simulink model "Simulation"  (R2021b)
settings: Solver=VariableStepAuto  StartTime=0.0  StopTime=10  RelTol=1e-3
values from neighbouring files (symbols this model uses):
  K1 = 3.38    [parameters.m]
  K2 = 0    [parameters.m]
  K3 = 63.96    [parameters.m]
  K4 = 0    [parameters.m]
  m = 30    [parameters.m]
  P = 1    [parameters.m]
  sinlamb = sind(70)    [parameters.m]
undefined symbols (not defined in the file or in its folder): sigbuilder_block
libraries: robotmobilelib x1
settings Model: Creator=DELL  LastModifiedBy=DELL

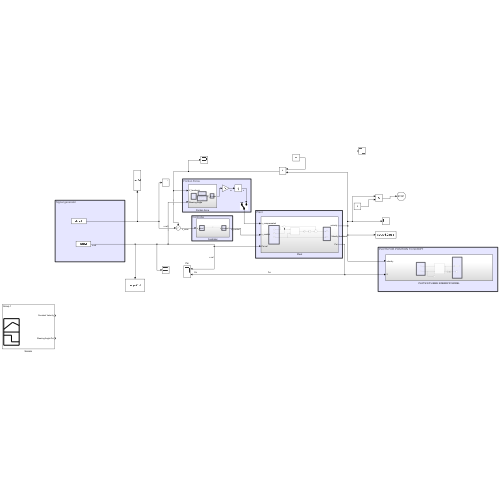
[thumbnail: Simulink's stored preview of the top-level diagram]
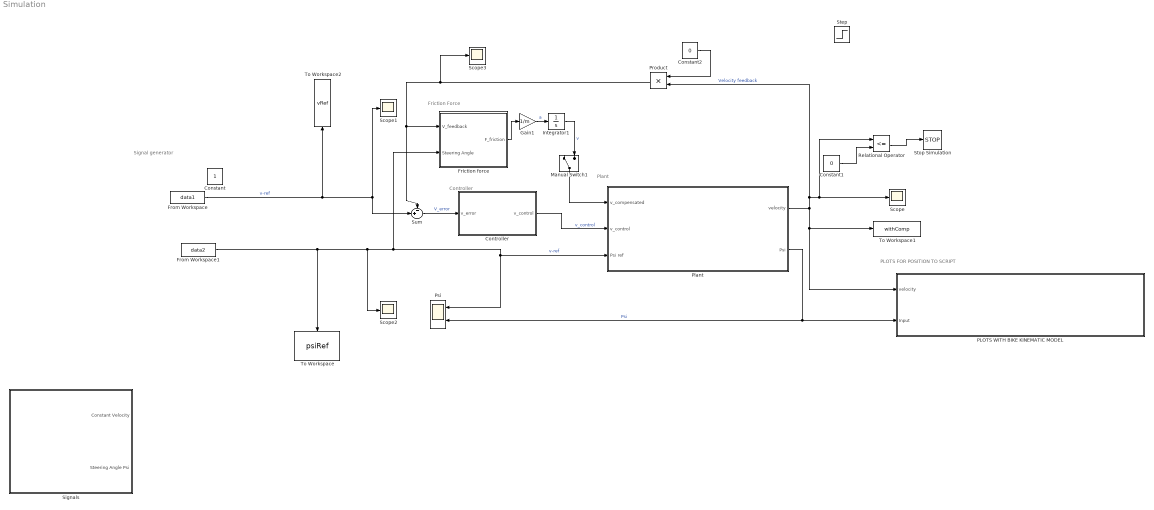
== system Simulation ==
  note: Plant
  note: Controller
  note: PLOTS FOR POSITION TO SCRIPT
  note: Signal generator
  note: Friction Force
  Constant1 : Constant  Value=0
  Constant2 : Constant  Value=0
  Controller : Subsystem
  Friction force : Subsystem
  From Workspace : FromWorkspace  VariableName=data1
  From Workspace1 : FromWorkspace  VariableName=data2
  Gain1 : Gain  Gain=1/m
  Integrator1 : Integrator
  Manual Switch1 : ManualSwitch
  PLOTS WITH BIKE KINEMATIC MODEL : Subsystem
  Plant : Subsystem
  Product : Product
  Psi : Scope  NumInputPorts=2
  Relational Operator : RelationalOperator  Operator=<=  OutDataTypeStr=boolean  RndMeth=Simplest
  Scope{,1..3} (4 alike) : Scope
  Signals : Subsystem  Tag=STV Subsys  LoadFcn=sigbuilder_block('load');  StartFcn=sigbuilder_block('start');  StopFcn=sigbuilder_block('stop');  ClipboardFcn=sigbuilder_block('clipboard');  mask(Sigbuilder block){tuvar=[0:10]}
      mask help: Simulink:masks:SigbuilderBlock_MD
      mask init:
      | if ~strcmp(get_param(bdroot(gcbh),'SimulationStatus'),'stopped') tuvar = sigbuilder_block('maskInit'); end
      settings: CopyFcn=sigbuilder_block('copy');  DeleteFcn=sigbuilder_block('delete');  ModelCloseFcn=sigbuilder_block('modelClose');  PreSaveFcn=sigbuilder_block('preSave');  PauseFcn=sigbuilder_block('pause');  ContinueFcn=sigbuilder_block('continue');  NameChangeFcn=sigbuilder_block('namechange');  OpenFcn=sigbuilder_block('open',[-17 64.5 550.5 362.5 ]);  CloseFcn=sigbuilder_block('close');
      mask Display: plot(0, 0, 100, 100,[2, 2, 32, 32, 2], [68, 8, 8, 68, 68],[32, 2], [38, 38], [32, 19, 2],[53, 60, 44], [32, 17, 17, 2],[16, 16, 31, 31]);txt = getActiveGroup(gcbh);text(2, 100, txt,'verticalAlignment', 'top');
  Step : Step  Time=5  Before=1  After=0  SampleTime=0
  Stop Simulation : Stop
  Sum : Sum  Inputs=-+|
  To Workspace : ToWorkspace  VariableName=psiRef  SaveFormat=Timeseries  SampleTime=-1
  To Workspace1 : ToWorkspace  VariableName=withComp  SaveFormat=Timeseries  SampleTime=-1
  To Workspace2 : ToWorkspace  VariableName=vRef  SaveFormat=Timeseries  SampleTime=-1
  Constant : Constant  IOType=siggen
  wires:
  From Workspace/1 -> To Workspace2/1, Sum/2, Scope1/1  "v-ref"
  Plant/1(velocity) -> Relational Operator/1, Scope/1, Product/2, To Workspace1/1, PLOTS WITH BIKE KINEMATIC MODEL/1(velocity)  "Velocity feedback"
  Plant/2(Psi) -> Psi/2, PLOTS WITH BIKE KINEMATIC MODEL/2(Input)  "Psi"
  Sum/1 -> Controller/1(v_error)  "V_error"
  Gain1/1 -> Integrator1/1  "a"
  Friction force/1(F_friction) -> Gain1/1
  Controller/1(v_control) -> Plant/2(v_control)  "v_control"
  Integrator1/1 -> Manual Switch1/2  "v"
  Manual Switch1/1 -> Plant/1(v_compensated)
  From Workspace1/1 -> Psi/1, Plant/3(Psi ref), Friction force/2(Steering Angle), Scope2/1, To Workspace/1  "v-ref"
  Constant1/1 -> Relational Operator/2
  Relational Operator/1 -> Stop Simulation/1
  Product/1 -> Scope3/1, Friction force/1(V_feedback), Sum/1
  Constant2/1 -> Product/1

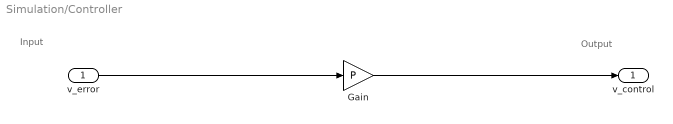
== system Simulation/Controller ==
  note: Output
  note: Input
  v_error : Inport
  Gain : Gain  Gain=P
  v_control : Outport
  wires:
  Gain/1 -> v_control/1
  v_error/1 -> Gain/1

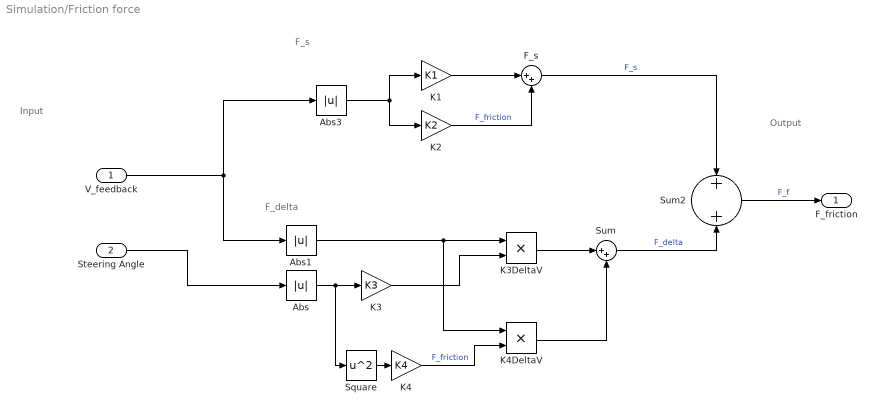
== system Simulation/Friction force ==
  note: F_delta
  note: Output
  note: Input
  note: F_s
  V_feedback : Inport
  Steering Angle : Inport  Port=2
  Abs : Abs
  Abs1 : Abs
  Abs3 : Abs
  F_s : Sum  Inputs=|++
  K1 : Gain  Gain=K1
  K2 : Gain  Gain=K2
  K3 : Gain  Gain=K3
  K3DeltaV : Product
  K4 : Gain  Gain=K4
  K4DeltaV : Product
  Square : Math  Operator=square  SaturateOnIntegerOverflow=on
  Sum : Sum  Inputs=|++
  Sum2 : Sum  Inputs=+|+
  F_friction : Outport
  wires:
  Square/1 -> K4/1
  K4DeltaV/1 -> Sum/2
  K3/1 -> K3DeltaV/2
  Abs1/1 -> K4DeltaV/1, K3DeltaV/1
  K4/1 -> K4DeltaV/2  "F_friction"
  K3DeltaV/1 -> Sum/1
  Abs/1 -> Square/1, K3/1
  Steering Angle/1 -> Abs/1
  F_s/1 -> Sum2/1  "F_s"
  K2/1 -> F_s/2  "F_friction"
  Abs3/1 -> K2/1, K1/1
  K1/1 -> F_s/1
  V_feedback/1 -> Abs1/1, Abs3/1
  Sum2/1 -> F_friction/1  "F_f"
  Sum/1 -> Sum2/2  "F_delta"

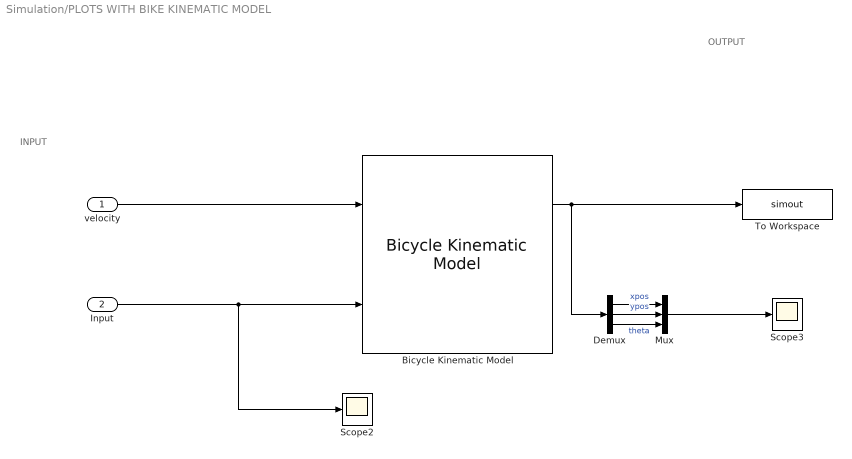
== system Simulation/PLOTS WITH BIKE KINEMATIC MODEL ==
  note: OUTPUT
  note: INPUT
  velocity : Inport
  Input : Inport  Port=2
  Bicycle Kinematic Model : robotmobilelib/Bicycle Kinematic Model  VehicleInputs=Vehicle Speed & Steering Angle  WheelBase=1.15  VehicleSpeedRange=[-100 100]  MaxSteeringAngle=pi/4  InitialState=[0; 0; 0]  SimulateUsing=Interpreted execution
      settings: SourceProductBaseCode=RO
  Demux : Demux  Outputs=3
  Mux : Mux  Inputs=3
  Scope2 : Scope
  Scope3 : Scope
  To Workspace : ToWorkspace  VariableName=simout  SaveFormat=Timeseries  SampleTime=-1
  wires:
  velocity/1 -> Bicycle Kinematic Model/1
  Input/1 -> Scope2/1, Bicycle Kinematic Model/2
  Demux/1 -> Mux/1  "xpos"
  Demux/2 -> Mux/2  "ypos"
  Demux/3 -> Mux/3  "theta"
  Mux/1 -> Scope3/1
  Bicycle Kinematic Model/1 -> Demux/1, To Workspace/1

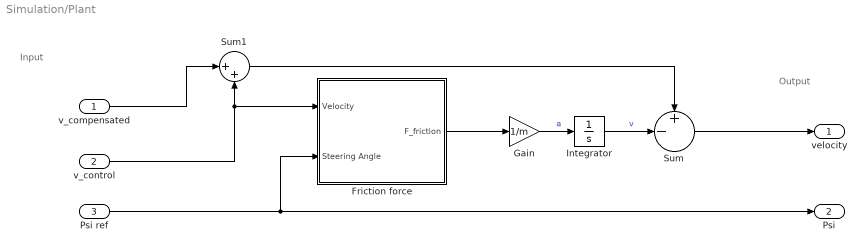
== system Simulation/Plant ==
  note: Output
  note: Input
  v_compensated : Inport
  v_control : Inport  Port=2
  Psi ref : Inport  Port=3
  Friction force : Subsystem
  Gain : Gain  Gain=1/m
  Integrator : Integrator
  Sum : Sum  Inputs=+-|
  Sum1 : Sum  Inputs=|++
  velocity : Outport
  Psi : Outport  Port=2
  wires:
  Psi ref/1 -> Friction force/2(Steering Angle), Psi/1
  Friction force/1(F_friction) -> Gain/1
  Gain/1 -> Integrator/1  "a"
  Integrator/1 -> Sum/2  "v"
  Sum/1 -> velocity/1
  v_compensated/1 -> Sum1/1
  v_control/1 -> Friction force/1(Velocity), Sum1/2
  Sum1/1 -> Sum/1

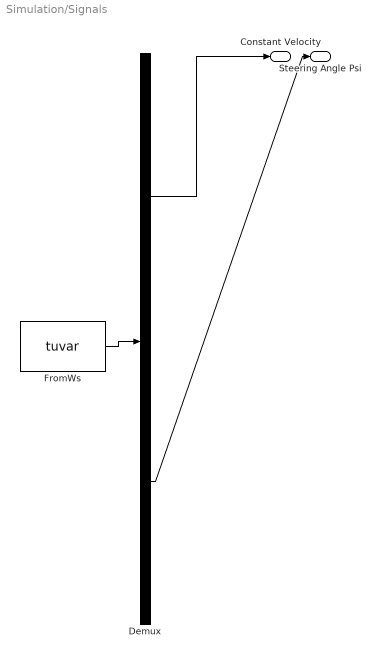
== system Simulation/Signals ==
  Demux : Demux  Tag=STV Demux  Outputs=2
      settings: DisplayOption=none
  FromWs : FromWorkspace  Tag=STV FromWs  VariableName=tuvar
      SigBuilderData=|
      | common.afterFinalStr = 'Extrapolate'
      | common.sampleTime = 0
      | dataSet.timeRange = [0 10]
      | dataSet.name = 'Group 1'
      | sbobj.Groups.Name = 'Group 1'
      | sbobj.Groups.Signals(1).Name = 'Constant Velocity'
      | sbobj.Groups.Signals(1).XData = [0 4 4 10]
      | sbobj.Groups.Signals(1).YData = [10 10 0 -0.1]
      | sbobj.Groups.Signals(2).Name = 'Steering Angle Psi'
      | sbobj.Groups.Signals(2).XData = [0 3 4 10]
      | sbobj.Groups.Signals(2).YData = [0 0 0.8 0.8]
  Constant Velocity : Outport  Tag=STV Outport
  Steering Angle Psi : Outport  Tag=STV Outport  Port=2
  wires:
  Demux/1 -> Constant Velocity/1
  FromWs/1 -> Demux/1
  Demux/2 -> Steering Angle Psi/1

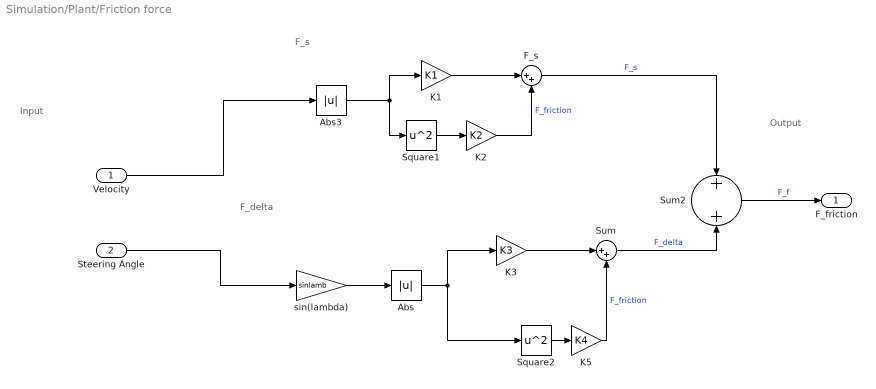
== system Simulation/Plant/Friction force ==
  note: F_delta
  note: Output
  note: Input
  note: F_s
  Velocity : Inport
  Steering Angle : Inport  Port=2
  Abs : Abs
  Abs3 : Abs
  F_s : Sum  Inputs=|++
  K1 : Gain  Gain=K1
  K2 : Gain  Gain=K2
  K3 : Gain  Gain=K3
  K5 : Gain  Gain=K4
  Square1 : Math  Operator=square  SaturateOnIntegerOverflow=on
  Square2 : Math  Operator=square  SaturateOnIntegerOverflow=on
  Sum : Sum  Inputs=|++
  Sum2 : Sum  Inputs=+|+
  sin(lambda) : Gain  Gain=sinlamb
  F_friction : Outport
  wires:
  Abs/1 -> Square2/1, K3/1
  K3/1 -> Sum/1
  F_s/1 -> Sum2/1  "F_s"
  K2/1 -> F_s/2  "F_friction"
  Abs3/1 -> K1/1, Square1/1
  K1/1 -> F_s/1
  Velocity/1 -> Abs3/1
  Sum2/1 -> F_friction/1  "F_f"
  Sum/1 -> Sum2/2  "F_delta"
  Square1/1 -> K2/1
  K5/1 -> Sum/2  "F_friction"
  Square2/1 -> K5/1
  sin(lambda)/1 -> Abs/1
  Steering Angle/1 -> sin(lambda)/1
